simulink model "RosToUdp"  (R2017b)
settings: Solver=VariableStepAuto  StartTime=0.0  StopTime=10.0  RelTol=1e-3
libraries: etargetslib x1, robotlib x1, dspnetwork x1
settings Model: Creator=antonio  LastModifiedBy=antonio

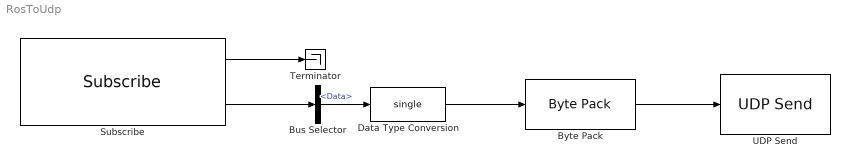
== system RosToUdp ==
  Bus Selector : BusSelector  OutputSignals=Data
  Byte Pack : etargetslib/Byte Pack  datatypes={'single'}  byteAlign=1
  Data Type Conversion : DataTypeConversion  OutDataTypeStr=single
  Subscribe : robotlib/Subscribe  SourceLibraryInfo=This block requires Robotics System Toolbox  topicSource=Select from ROS network  topic=/left_hand/position_curr  messageType=std_msgs/Float64  sampleTime=0.01  messageQueueLength=1
      settings: SourceProductBaseCode=RO
  Terminator : Terminator
  UDP Send : dspnetwork/UDP Send  remoteURL='10.24.4.10'  remotePort=16106  localURL='0.0.0.0'  localPortSource=Automatically determine  localPort=-1  sampletime=-1  blockPlatform=HOST  separateLengthPort=0
      settings: SourceProductName=DSP System Toolbox  SourceProductBaseCode=DS
  wires:
  Subscribe/1 -> Terminator/1
  Subscribe/2 -> Bus Selector/1
  Bus Selector/1 -> Data Type Conversion/1  "<Data>"
  Data Type Conversion/1 -> Byte Pack/1
  Byte Pack/1 -> UDP Send/1
